simulink subsystem "Transmitter"  (R2022b)
settings: Solver=VariableStepAuto  StartTime=0.0  StopTime=10.0  RelTol=1e-3
undefined symbols (not defined in the file or in its folder): debugHeaderGain, G, Rsym
libraries: simulink x44, hdlsllib x29, dspsigops x7, dsphdlfiltering2 x1, whdlmod x1
(part 1 of 2)
settings Model: Creator=svdvl  LastModifiedBy=svdvl

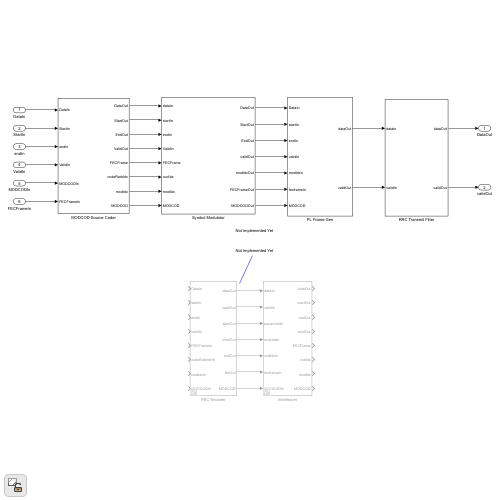
[thumbnail: Simulink's stored preview of the top-level diagram]
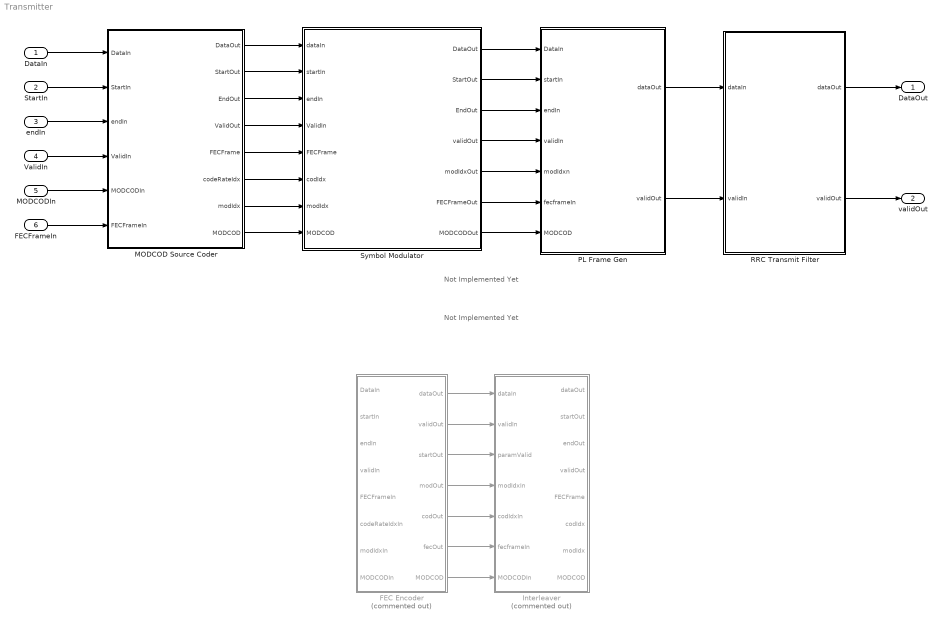
== system Transmitter ==
  note: Not Implemented Yet
  note: Not Implemented Yet
  DataIn : Inport
  StartIn : Inport  Port=2
  endIn : Inport  Port=3
  ValidIn : Inport  Port=4
  MODCODIn : Inport  Port=5
  FECFrameIn : Inport  Port=6
  FEC Encoder : Subsystem  Commented=on
  Interleaver : Subsystem  Commented=on
  MODCOD Source Coder : Subsystem
  PL Frame Gen : Subsystem
  RRC Transmit Filter : Subsystem
  Symbol Modulator : Subsystem
  DataOut : Outport
  validOut : Outport  Port=2
  wires:
  RRC Transmit Filter/2(validOut) -> validOut/1
  RRC Transmit Filter/1(dataOut) -> DataOut/1
  MODCOD Source Coder/5(FECFrame) -> Symbol Modulator/5(FECFrame)
  MODCOD Source Coder/3(EndOut) -> Symbol Modulator/3(endIn)
  MODCOD Source Coder/8(MODCOD) -> Symbol Modulator/8(MODCOD)
  MODCOD Source Coder/6(codeRateIdx) -> Symbol Modulator/6(codIdx)
  MODCOD Source Coder/4(ValidOut) -> Symbol Modulator/4(ValidIn)
  MODCOD Source Coder/2(StartOut) -> Symbol Modulator/2(startIn)
  MODCOD Source Coder/1(DataOut) -> Symbol Modulator/1(dataIn)
  Symbol Modulator/6(FECFrameOut) -> PL Frame Gen/6(fecframeIn)
  MODCOD Source Coder/7(modIdx) -> Symbol Modulator/7(modIdx)
  endIn/1 -> MODCOD Source Coder/3(endIn)
  Symbol Modulator/2(StartOut) -> PL Frame Gen/2(startIn)
  Symbol Modulator/7(MODCODOut) -> PL Frame Gen/7(MODCOD)
  StartIn/1 -> MODCOD Source Coder/2(StartIn)
  FECFrameIn/1 -> MODCOD Source Coder/6(FECFrameIn)
  PL Frame Gen/1(dataOut) -> RRC Transmit Filter/1(dataIn)
  DataIn/1 -> MODCOD Source Coder/1(DataIn)
  MODCODIn/1 -> MODCOD Source Coder/5(MODCODIn)
  Symbol Modulator/3(EndOut) -> PL Frame Gen/3(endIn)
  Symbol Modulator/5(modIdxOut) -> PL Frame Gen/5(modIdxn)
  Symbol Modulator/1(DataOut) -> PL Frame Gen/1(DataIn)
  Symbol Modulator/4(validOut) -> PL Frame Gen/4(validIn)
  PL Frame Gen/2(validOut) -> RRC Transmit Filter/2(validIn)
  ValidIn/1 -> MODCOD Source Coder/4(ValidIn)
  FEC Encoder/7(MODCOD) -> Interleaver/7(MODCODIn)
  FEC Encoder/1(dataOut) -> Interleaver/1(dataIn)
  FEC Encoder/4(modOut) -> Interleaver/4(modIdxIn)
  FEC Encoder/5(codOut) -> Interleaver/5(codIdxIn)
  FEC Encoder/3(startOut) -> Interleaver/3(paramValid)
  FEC Encoder/2(validOut) -> Interleaver/2(validIn)
  FEC Encoder/6(fecOut) -> Interleaver/6(fecframeIn)

== system Transmitter/FEC Encoder ==
  DataIn : Inport
  startIn : Inport  Port=2
  endIn : Inport  Port=3
  validIn : Inport  Port=4
  FECFrameIn : Inport  Port=5
  codeRateIdxIn : Inport  Port=6
  modIdxIn : Inport  Port=7
  MODCODIn : Inport  Port=8
  Terminator : Terminator
  dataOut : Outport
  validOut : Outport  Port=2
  startOut : Outport  Port=3
  modOut : Outport  Port=4
  codOut : Outport  Port=5
  fecOut : Outport  Port=6
  MODCOD : Outport  Port=7
  wires:
  DataIn/1 -> dataOut/1
  startIn/1 -> startOut/1
  modIdxIn/1 -> modOut/1
  codeRateIdxIn/1 -> codOut/1
  FECFrameIn/1 -> fecOut/1
  MODCODIn/1 -> MODCOD/1
  validIn/1 -> validOut/1
  endIn/1 -> Terminator/1

== system Transmitter/Interleaver ==
  dataIn : Inport
  validIn : Inport  Port=2
  paramValid : Inport  Port=3
  modIdxIn : Inport  Port=4
  codIdxIn : Inport  Port=5
  fecframeIn : Inport  Port=6
  MODCODIn : Inport  Port=7
  dataOut : Outport
  startOut : Outport  Port=2
  endOut : Outport  Port=3
  validOut : Outport  Port=4
  FECFrame : Outport  Port=5
  codIdx : Outport  Port=6
  modIdx : Outport  Port=7
  MODCOD : Outport  Port=8
  wires:
  dataIn/1 -> dataOut/1
  validIn/1 -> validOut/1

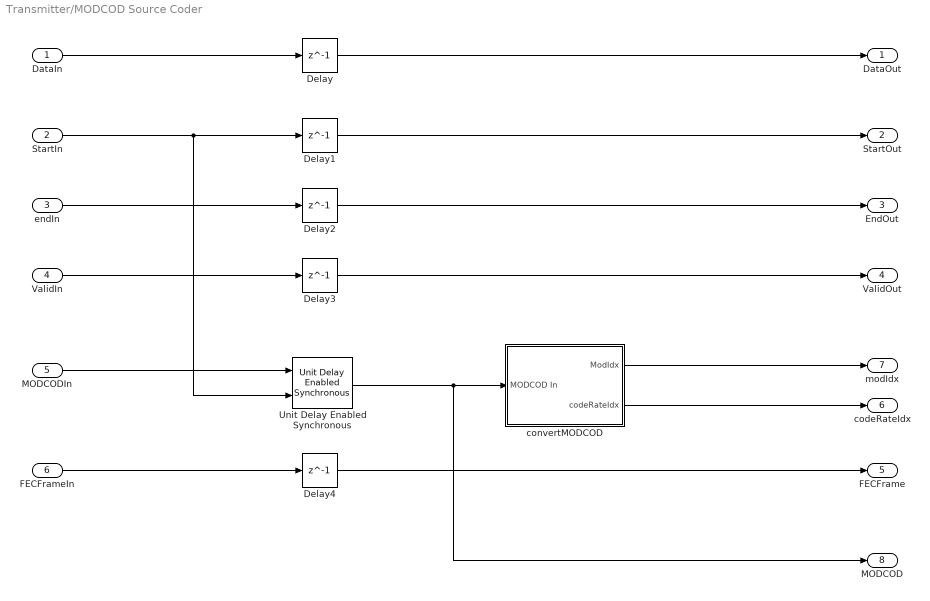
== system Transmitter/MODCOD Source Coder ==
  DataIn : Inport
  StartIn : Inport  Port=2
  endIn : Inport  Port=3
  ValidIn : Inport  Port=4
  MODCODIn : Inport  Port=5
  FECFrameIn : Inport  Port=6
  Delay{,1..4} (5 alike) : Delay  DelayLength=1
  Unit Delay Enabled Synchronous : hdlsllib/Discrete/Unit Delay Enabled Synchronous  InitialCondition=0.0  SampleTime=-1
  convertMODCOD : Subsystem
  DataOut : Outport
  StartOut : Outport  Port=2
  EndOut : Outport  Port=3
  ValidOut : Outport  Port=4
  FECFrame : Outport  Port=5
  codeRateIdx : Outport  Port=6
  modIdx : Outport  Port=7
  MODCOD : Outport  Port=8
  wires:
  MODCODIn/1 -> Unit Delay Enabled Synchronous/1
  DataIn/1 -> Delay/1
  StartIn/1 -> Unit Delay Enabled Synchronous/2, Delay1/1
  endIn/1 -> Delay2/1
  ValidIn/1 -> Delay3/1
  Unit Delay Enabled Synchronous/1 -> convertMODCOD/1(MODCOD In), MODCOD/1
  convertMODCOD/1(ModIdx) -> modIdx/1
  convertMODCOD/2(codeRateIdx) -> codeRateIdx/1
  FECFrameIn/1 -> Delay4/1
  Delay/1 -> DataOut/1
  Delay1/1 -> StartOut/1
  Delay2/1 -> EndOut/1
  Delay3/1 -> ValidOut/1
  Delay4/1 -> FECFrame/1

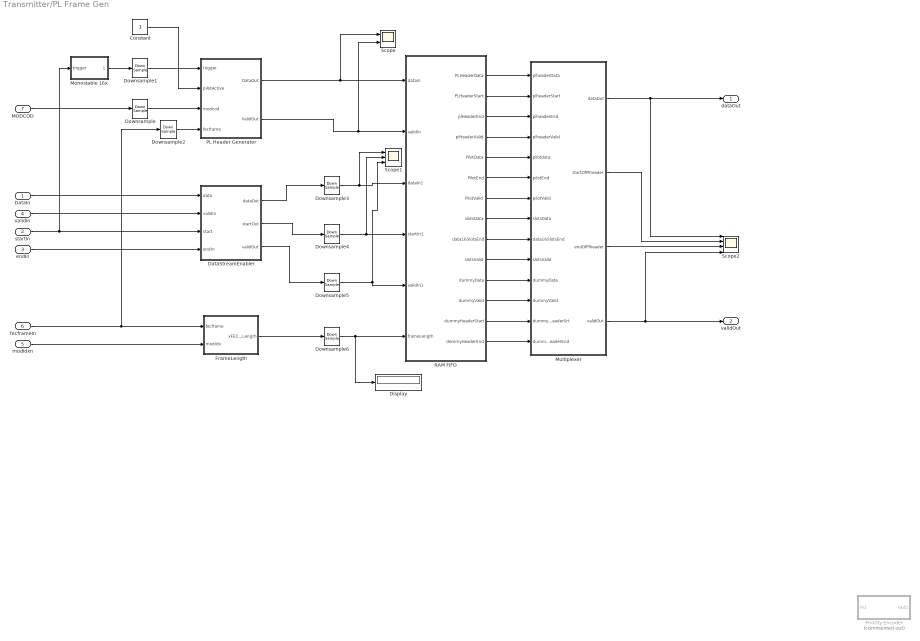
== system Transmitter/PL Frame Gen ==
  DataIn : Inport
  startIn : Inport  Port=2
  endIn : Inport  Port=3
  validIn : Inport  Port=4
  modIdxn : Inport  Port=5
  fecframeIn : Inport  Port=6
  MODCOD : Inport  Port=7
  Constant : Constant  OutDataTypeStr=boolean  SampleTime=2/Rsym
  DataStreamEnabler : Subsystem
  Display : Display
  Downsample : DownSample  N=16  RateOptions=Allow multirate processing
  Downsample1 : DownSample  N=16  RateOptions=Allow multirate processing
  Downsample2 : DownSample  N=16  RateOptions=Allow multirate processing
  Downsample{3..6} (4 alike) : DownSample  N=8  RateOptions=Allow multirate processing
  FrameLength : Subsystem
  Monostable 16x : Subsystem
  Multiplexer : Subsystem
  PL Header Generator : Subsystem
  Priority Encoder : Subsystem  Commented=on
  RAM FIFO : Subsystem
  Scope : Scope  NumInputPorts=2
  Scope1 : Scope  NumInputPorts=3
  Scope2 : Scope  NumInputPorts=4
  dataOut : Outport
  validOut : Outport  Port=2
  wires:
  MODCOD/1 -> Downsample/1
  Downsample/1 -> PL Header Generator/3(modcod)
  startIn/1 -> DataStreamEnabler/3(start), Monostable 16x/1(trigger)
  DataIn/1 -> DataStreamEnabler/1(data)
  validIn/1 -> DataStreamEnabler/2(validIn)
  endIn/1 -> DataStreamEnabler/4(endIn)
  fecframeIn/1 -> Downsample2/1, FrameLength/1(fecframe)
  modIdxn/1 -> FrameLength/2(modIdx)
  Downsample1/1 -> PL Header Generator/1(trigger)
  Downsample2/1 -> PL Header Generator/4(fecframe)
  DataStreamEnabler/1(dataOut) -> Downsample3/1
  DataStreamEnabler/2(startOut) -> Downsample4/1
  DataStreamEnabler/3(validOut) -> Downsample5/1
  FrameLength/1(xFECFrameLength) -> Downsample6/1
  Constant/1 -> PL Header Generator/2(pilotActive)
  Downsample6/1 -> Display/1, RAM FIFO/6(frameLength)
  PL Header Generator/1(DataOut) -> Scope/1, RAM FIFO/1(dataIn)
  PL Header Generator/2(ValidOut) -> Scope/2, RAM FIFO/2(validIn)
  Downsample3/1 -> Scope1/1, RAM FIFO/3(dataIn1)
  Downsample4/1 -> Scope1/2, RAM FIFO/4(startIn1)
  Downsample5/1 -> Scope1/3, RAM FIFO/5(validIn1)
  Monostable 16x/1(validOut) -> Downsample1/1
  RAM FIFO/1(PLHeaderData) -> Multiplexer/1(plheaderData)
  RAM FIFO/2(PLHeaderStart) -> Multiplexer/2(plheaderStart)
  RAM FIFO/3(plHeaderEnd) -> Multiplexer/3(plheaderEnd)
  RAM FIFO/4(plHeaderValid) -> Multiplexer/4(plheaderValid)
  RAM FIFO/5(PilotData) -> Multiplexer/5(pilotdata)
  RAM FIFO/6(PilotEnd) -> Multiplexer/6(pilotEnd)
  RAM FIFO/7(PilotValid) -> Multiplexer/7(pilotValid)
  RAM FIFO/8(slotsData) -> Multiplexer/8(slotsData)
  RAM FIFO/9(data16SlotsEnd) -> Multiplexer/9(data16SlotsEnd)
  RAM FIFO/10(slotsValid) -> Multiplexer/10(slotsValid)
  RAM FIFO/11(dummyData) -> Multiplexer/11(dummyData)
  RAM FIFO/12(dummyValid) -> Multiplexer/12(dummyValid)
  RAM FIFO/13(dummyHeaderStart) -> Multiplexer/13(dummyHeaderSrt)
  RAM FIFO/14(demmyHeaderEnd) -> Multiplexer/14(dummyHeaderEnd)
  Multiplexer/1(dataOut) -> dataOut/1, Scope2/1
  Multiplexer/2(startOfPlheader) -> Scope2/2
  Multiplexer/3(endOfPlheader) -> Scope2/3
  Multiplexer/4(validOut) -> validOut/1, Scope2/4

== system Transmitter/RRC Transmit Filter ==
  dataIn : Inport
  validIn : Inport  Port=2
  Discrete FIR Filter : dsphdlfiltering2/Discrete FIR Filter  NumeratorSource=Property  Numerator="[-0.00285820997079789\t0.00137733032508190\t0.00315455482520775\t-0.00356415296709377\t-0.00206211933009069\t0.00514477794743620\t-0.000825518525453186\t-0.00481272795526686\t0.00560922270003514\t0.000910808542107733\t-0.0120044818773511\t0.00862996822246556\t0.0193455321229390\t-0.0268242332250627\t-0.0266806119948057\t0.0600224093867556\t0.0329422984385442\t-0.130628932045810\t-0.0371565869289195\t0.443442194227448\t0.745765109300838\t0.443442194227448\t-0.0371565869289195\t-0.130628932045810\t0.0329422984385442\t0.0600224093867556\t-0.0266806119948057\t-0.0268242332250627\t0.0193455321229390\t0.00862996822246556\t-0.0120044818773511\t0.000910808542107733\t0.00560922270003514\t-0.00481272795526686\t-0.000825518525453186\t0.00514477794743620\t-0.00206211933009069\t-0.00356415296709377\t0.00315455482520775\t0.00137733032508190\t-0.00285820997079789]"  NumeratorPrototype=[]  FilterStructure=Direct form systolic  SerializationOption=Minimum number of cycles between valid input samples  NumCycles=2  NumberOfMultipliers=2  SimulateUsing=Code generation  roundingMode=Floor  overflowMode=off  CoefficientsDataTypeStr=Inherit: Same word length as input  OutputDataTypeStr=Inherit: Same word length as input  ResetInputPort=off  HDLGlobalReset=off
  Repeat : dspsigops/Repeat  N=2  RateOptions=Allow multirate processing  ic=0  mode=Unused parameter value
      settings: LibrarySourceBlock=dsphdlsupportsigops/Repeat
  Upsample : dspsigops/Upsample  N=2  phase=0  RateOptions=Allow multirate processing  ic=0  mode=Unused parameter value
      settings: LibrarySourceBlock=dsphdlsupportsigops/Upsample
  dataOut : Outport
  validOut : Outport  Port=2
  wires:
  dataIn/1 -> Upsample/1
  Discrete FIR Filter/1 -> dataOut/1
  Discrete FIR Filter/2 -> validOut/1
  validIn/1 -> Repeat/1
  Upsample/1 -> Discrete FIR Filter/1
  Repeat/1 -> Discrete FIR Filter/2

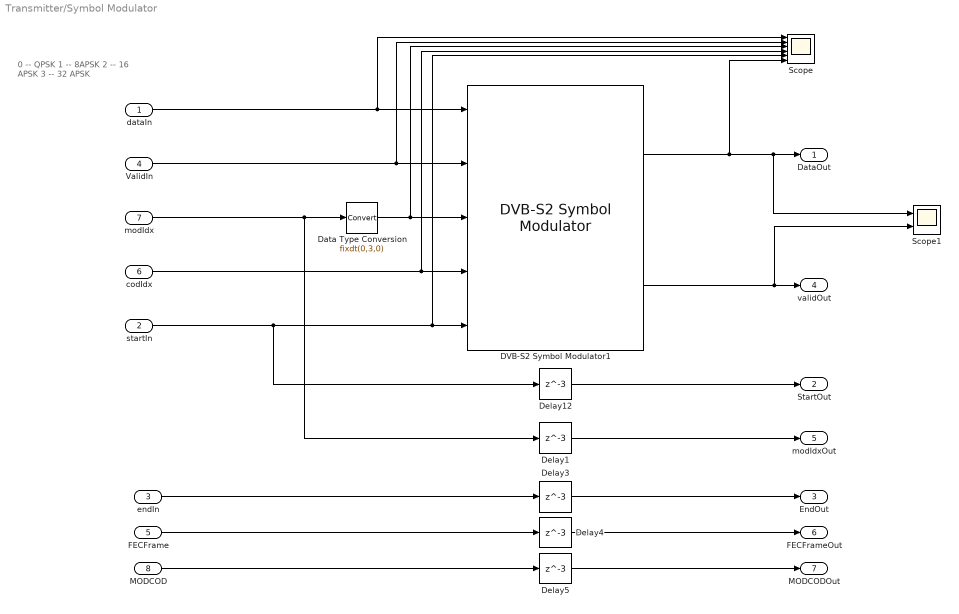
== system Transmitter/Symbol Modulator ==
  note: 0 -- QPSK
      | 1 -- 8APSK
      | 2 -- 16 APSK
      | 3 -- 32 APSK
  dataIn : Inport
  startIn : Inport  Port=2
  endIn : Inport  Port=3
  ValidIn : Inport  Port=4
  FECFrame : Inport  Port=5
  codIdx : Inport  Port=6
  modIdx : Inport  Port=7
  MODCOD : Inport  Port=8
  DVB-S2 Symbol Modulator1 : whdlmod/DVB-S2 Symbol Modulator  ModulationSourceParams=Input port  ModulationScheme=QPSK  CodeRateAPSK=3/4  UnitAveragePower=on  SimulateUsing=Code generation  OutputDataType=double  WordLength=18
  Data Type Conversion : DataTypeConversion  OutDataTypeStr=fixdt(0,3,0)  SaturateOnIntegerOverflow=off  RndMeth=Floor
  Delay{1,3..5,12} (5 alike) : Delay  DelayLength=3
  Scope : Scope  NumInputPorts=6
  Scope1 : Scope  NumInputPorts=2
  DataOut : Outport
  StartOut : Outport  Port=2
  EndOut : Outport  Port=3
  validOut : Outport  Port=4
  modIdxOut : Outport  Port=5
  FECFrameOut : Outport  Port=6
  MODCODOut : Outport  Port=7
  wires:
  dataIn/1 -> Scope/1, DVB-S2 Symbol Modulator1/1
  ValidIn/1 -> Scope/2, DVB-S2 Symbol Modulator1/2
  modIdx/1 -> Delay1/1, Data Type Conversion/1
  codIdx/1 -> Scope/4, DVB-S2 Symbol Modulator1/4
  startIn/1 -> Delay12/1, Scope/5, DVB-S2 Symbol Modulator1/5
  Data Type Conversion/1 -> Scope/3, DVB-S2 Symbol Modulator1/3
  DVB-S2 Symbol Modulator1/1 -> Scope/6, Scope1/1, DataOut/1
  DVB-S2 Symbol Modulator1/2 -> Scope1/2, validOut/1
  FECFrame/1 -> Delay4/1
  MODCOD/1 -> Delay5/1
  endIn/1 -> Delay3/1
  Delay12/1 -> StartOut/1
  Delay1/1 -> modIdxOut/1
  Delay3/1 -> EndOut/1
  Delay4/1 -> FECFrameOut/1
  Delay5/1 -> MODCODOut/1

== system Transmitter/MODCOD Source Coder/convertMODCOD ==
  note: 0 -- 1/4
      | 1 -- 1/3
      | 2 -- 2/5
      | 3 -- 1/2
      | 4 -- 3/5
      | 5 -- 2/3
      | 6 -- 3/4
      | 7 -- 4/5
      | 8 -- 5/6
      | 9 -- 8/9
      | 10 -- 9/10
  note: 0 -- QPSK
      | 1 -- 8APSK
      | 2 -- 16 APSK
      | 3 -- 32 APSK
  note: MODCOD DVB-S2
      | 1-11 QPSK
      | 2-17 8APSK
      | 18-23 16 APSK
      | 24-28 32 APSK
      | 29 QPSK (1/2) NEW
      | 29-31 RESERVED
      | 32 DUMMY
  MODCOD In : Inport
  1-D Lookup Table : Lookup_n-D  NumberOfTableDimensions=1  BreakpointsSpecification=Even spacing  BreakpointsForDimension1=[1:29]  Table=[0, 1, 2, 3, 4, 5, 6, 7, 8, 9, 10, 4, 5, 6, 8, 9, 10, 5, 6, 7, 8, 9, 10, 6, 7, 8, 9, 10, 3]  ExtrapMethod=Clip  UseLastTableValue=on  InternalRulePriority=Speed  OutDataTypeStr=fixdt(0, 4, 0)  RndMeth=Simplest
  Compare To Constant : simulink/Logic and Bit Operations/Compare To Constant  relop=<  const=12  OutDataTypeStr=boolean
  Compare To Constant1 : simulink/Logic and Bit Operations/Compare To Constant  relop=<  const=18  OutDataTypeStr=boolean
  Compare To Constant2 : simulink/Logic and Bit Operations/Compare To Constant  relop=<  const=24  OutDataTypeStr=boolean
  Compare To Constant3 : simulink/Logic and Bit Operations/Compare To Constant  relop===  const=29  OutDataTypeStr=boolean
  Constant : Constant  Value=0  OutDataTypeStr=fixdt(0,3,0)  SampleTime=-1
  Constant1 : Constant  OutDataTypeStr=fixdt(0,3,0)  SampleTime=-1
  Constant2 : Constant  Value=2  OutDataTypeStr=fixdt(0,3,0)  SampleTime=-1
  Constant3 : Constant  Value=3  OutDataTypeStr=fixdt(0,3,0)  SampleTime=-1
  Logical Operator : Logic  Operator=OR  AllPortsSameDT=off  OutDataTypeStr=boolean
  Scope : Scope  NumInputPorts=2
  Switch : Switch  Criteria=u2 ~= 0  SaturateOnIntegerOverflow=off  InputSameDT=off
  Switch1 : Switch  Criteria=u2 ~= 0  SaturateOnIntegerOverflow=off  InputSameDT=off
  Switch2 : Switch  Criteria=u2 ~= 0  SaturateOnIntegerOverflow=off  InputSameDT=off
  ModIdx : Outport
  codeRateIdx : Outport  Port=2
  wires:
  Constant3/1 -> Switch2/3
  Compare To Constant/1 -> Switch/2
  Constant1/1 -> Switch1/1
  Compare To Constant1/1 -> Switch1/2
  Switch/1 -> Scope/1, ModIdx/1
  MODCOD In/1 -> Compare To Constant1/1, Compare To Constant/1, Compare To Constant3/1, 1-D Lookup Table/1, Compare To Constant2/1
  Constant/1 -> Switch/1
  Constant2/1 -> Switch2/1
  Switch2/1 -> Switch1/3
  Switch1/1 -> Switch/3
  1-D Lookup Table/1 -> Scope/2, codeRateIdx/1
  Compare To Constant2/1 -> Logical Operator/1
  Compare To Constant3/1 -> Logical Operator/2
  Logical Operator/1 -> Switch2/2

== system Transmitter/PL Frame Gen/DataStreamEnabler ==
  data : Inport
  validIn : Inport  Port=2
  start : Inport  Port=3
  endIn : Inport  Port=4
  Scope : Scope  NumInputPorts=3
  Unit Delay Enabled Synchronous : hdlsllib/Discrete/Unit Delay Enabled Synchronous  InitialCondition=0.0  SampleTime=-1
  monostable 8x : Subsystem
  dataOut : Outport
  startOut : Outport  Port=2
  validOut : Outport  Port=3
  wires:
  data/1 -> Unit Delay Enabled Synchronous/1
  validIn/1 -> Unit Delay Enabled Synchronous/2
  Unit Delay Enabled Synchronous/1 -> Scope/1, dataOut/1
  start/1 -> monostable 8x/1(startIn)
  endIn/1 -> monostable 8x/2(endIn)
  monostable 8x/1(startOut) -> Scope/2, startOut/1
  monostable 8x/2(ValidOut) -> Scope/3, validOut/1

== system Transmitter/PL Frame Gen/FrameLength ==
  note: Number of symbols in a frame
  note: 0 normal frame
      | 1 short frame
      | 2 medium frame
  note: modIdx encodes the number of bits in a symbol
      | 0 -- 2 bits per constellation point
      | 1 -- 3 bits
      | 2 -- 4 bits
      | 3 -- 5 bits
      | 4 -- 6 bits
  fecframe : Inport
  modIdx : Inport  Port=2
  Display : Display
  Display1 : Display
  Display2 : Display
  Medium Frame xFECFrame Length1 : Lookup_n-D  NumberOfTableDimensions=1  BreakpointsSpecification=Even spacing  BreakpointsForDimension1=[-5:5]  BreakpointsForDimension1FirstPoint=0  Table=32400./log2([4 8 16 32 64])  TableDataTypeStr=fixdt(0,15,0)  InterpMethod=Flat  InternalRulePriority=Speed  OutDataTypeStr=fixdt(0,15,0)  RndMeth=Simplest
  Multiport Switch : MultiPortSwitch  DataPortOrder=Zero-based contiguous  zeroidx=on  SaturateOnIntegerOverflow=off  InputSameDT=off
  Normal Frame xFECFrame Length : Lookup_n-D  NumberOfTableDimensions=1  BreakpointsSpecification=Even spacing  BreakpointsForDimension1=[-5:5]  BreakpointsForDimension1FirstPoint=0  Table=64800./log2([4 8 16 32 64])  TableDataTypeStr=fixdt(0,15,0)  InterpMethod=Flat  InternalRulePriority=Speed  OutDataTypeStr=fixdt(0,15,0)  RndMeth=Simplest
  Short Frame xFECFrame Length : Lookup_n-D  NumberOfTableDimensions=1  BreakpointsSpecification=Even spacing  BreakpointsForDimension1=[-5:5]  BreakpointsForDimension1FirstPoint=0  Table=16200./log2([4 8 16 32 64])  TableDataTypeStr=fixdt(0,15,0)  InterpMethod=Flat  InternalRulePriority=Speed  OutDataTypeStr=fixdt(0,15,0)  RndMeth=Simplest
  xFECFrameLength : Outport
  wires:
  fecframe/1 -> Multiport Switch/1, Display/1
  Normal Frame xFECFrame Length/1 -> Multiport Switch/2
  Multiport Switch/1 -> xFECFrameLength/1, Display1/1
  modIdx/1 -> Medium Frame xFECFrame Length1/1, Short Frame xFECFrame Length/1, Normal Frame xFECFrame Length/1, Display2/1
  Medium Frame xFECFrame Length1/1 -> Multiport Switch/4
  Short Frame xFECFrame Length/1 -> Multiport Switch/3

== system Transmitter/PL Frame Gen/Monostable 16x ==
  trigger : Inport
  Compare To Constant : simulink/Logic and Bit Operations/Compare To Constant  relop===  const=16  OutDataTypeStr=boolean
  Compare To Constant1 : simulink/Logic and Bit Operations/Compare To Constant  relop=~=  const=0  OutDataTypeStr=boolean
  HDL Counter : hdlsllib/Sources/HDL Counter  CountType=Count limited  CountInit=0  CountStep=1  CountMax=16  CountFromType=Initial value  CountFrom=0  CountResetPort=on  CountLoadPort=off  CountEnbPort=on  CountDirPort=off  CountHitOutputPort=off  CountDataType=Unsigned  CountWordLen=8  CountFracLen=0  CountSampTime=1
  Logical Operator : Logic  Operator=OR  AllPortsSameDT=off  OutDataTypeStr=boolean
  Scope : Scope  NumInputPorts=3
  validOut : Outport
  wires:
  HDL Counter/1 -> Scope/1, Compare To Constant1/1, Compare To Constant/1
  trigger/1 -> Logical Operator/1
  Logical Operator/1 -> Scope/2, HDL Counter/2
  Compare To Constant/1 -> HDL Counter/1, Scope/3
  Compare To Constant1/1 -> Logical Operator/2, validOut/1

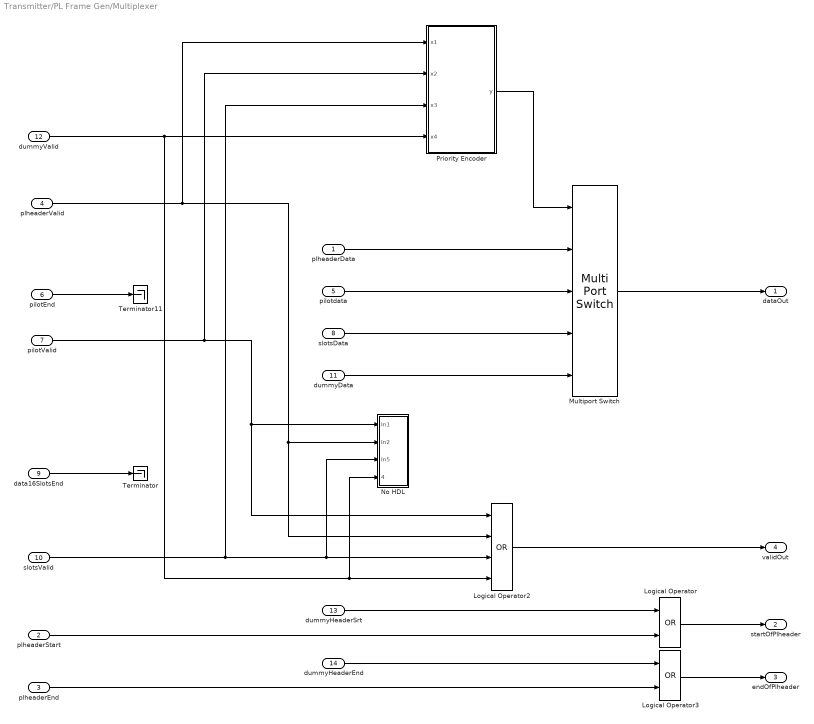
== system Transmitter/PL Frame Gen/Multiplexer ==
  plheaderData : Inport
  plheaderStart : Inport  Port=2
  plheaderEnd : Inport  Port=3
  plheaderValid : Inport  Port=4
  pilotdata : Inport  Port=5
  pilotEnd : Inport  Port=6
  pilotValid : Inport  Port=7
  slotsData : Inport  Port=8
  data16SlotsEnd : Inport  Port=9
  slotsValid : Inport  Port=10
  dummyData : Inport  Port=11
  dummyValid : Inport  Port=12
  dummyHeaderSrt : Inport  Port=13
  dummyHeaderEnd : Inport  Port=14
  Logical Operator : Logic  Operator=OR  AllPortsSameDT=off  OutDataTypeStr=boolean
  Logical Operator2 : Logic  Operator=OR  Inputs=4  AllPortsSameDT=off  OutDataTypeStr=boolean
  Logical Operator3 : Logic  Operator=OR  AllPortsSameDT=off  OutDataTypeStr=boolean
  Multiport Switch : MultiPortSwitch  DataPortOrder=Zero-based contiguous  Inputs=4  zeroidx=on  SaturateOnIntegerOverflow=off  InputSameDT=off
  No HDL : Subsystem
  Priority Encoder : MATLAB Function  TreatAsAtomicUnit=on
  Terminator : Terminator
  Terminator11 : Terminator
  dataOut : Outport
  startOfPlheader : Outport  Port=2
  endOfPlheader : Outport  Port=3
  validOut : Outport  Port=4
  wires:
  slotsValid/1 -> Priority Encoder/3(x3), No HDL/3(In5), Logical Operator2/3
  pilotValid/1 -> Priority Encoder/2(x2), Logical Operator2/1, No HDL/1(In1)
  data16SlotsEnd/1 -> Terminator/1
  plheaderValid/1 -> Priority Encoder/1(x1), Logical Operator2/2, No HDL/2(In2)
  pilotEnd/1 -> Terminator11/1
  Logical Operator2/1 -> validOut/1
  plheaderStart/1 -> Logical Operator/2
  dummyValid/1 -> No HDL/4(dummyValid), Logical Operator2/4, Priority Encoder/4(x4)
  Priority Encoder/1(y) -> Multiport Switch/1
  Multiport Switch/1 -> dataOut/1
  plheaderEnd/1 -> Logical Operator3/2
  plheaderData/1 -> Multiport Switch/2
  pilotdata/1 -> Multiport Switch/3
  slotsData/1 -> Multiport Switch/4
  dummyData/1 -> Multiport Switch/5
  dummyHeaderSrt/1 -> Logical Operator/1
  dummyHeaderEnd/1 -> Logical Operator3/1
  Logical Operator/1 -> startOfPlheader/1
  Logical Operator3/1 -> endOfPlheader/1

== system Transmitter/PL Frame Gen/PL Header Generator ==
  note: 1 at the start of the frame, else zero
  trigger : Inport
  pilotActive : Inport  Port=2
  modcod : Inport  Port=3
  fecframe : Inport  Port=4
  PL Header Bits Generator : Subsystem
  Terminator : Terminator
  Terminator1 : Terminator
  pi2 BSPK Modulator : Subsystem
  DataOut : Outport
  ValidOut : Outport  Port=2
  wires:
  modcod/1 -> PL Header Bits Generator/3(modcod)
  fecframe/1 -> PL Header Bits Generator/4(fecframe)
  pilotActive/1 -> PL Header Bits Generator/2(pilotActive)
  PL Header Bits Generator/1(bitsOut) -> pi2 BSPK Modulator/1(bitsIn)
  PL Header Bits Generator/5(UnscrambledBits) -> Terminator1/1
  PL Header Bits Generator/2(bitsStart) -> pi2 BSPK Modulator/2(startIn)
  PL Header Bits Generator/3(bitsEnd) -> Terminator/1
  PL Header Bits Generator/4(bitsValid) -> pi2 BSPK Modulator/3(validIn)
  trigger/1 -> PL Header Bits Generator/1(trigger)
  pi2 BSPK Modulator/1(dataOut) -> DataOut/1
  pi2 BSPK Modulator/2(validOut) -> ValidOut/1

== system Transmitter/PL Frame Gen/Priority Encoder ==
  In1 : Inport
  Out1 : Outport
  wires:
  In1/1 -> Out1/1

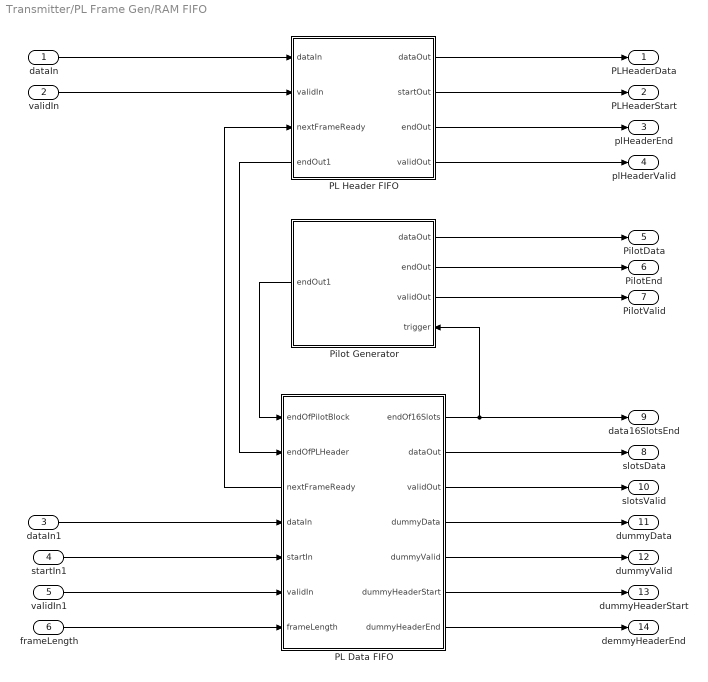
== system Transmitter/PL Frame Gen/RAM FIFO ==
  dataIn : Inport
  validIn : Inport  Port=2
  dataIn1 : Inport  Port=3
  startIn1 : Inport  Port=4
  validIn1 : Inport  Port=5
  frameLength : Inport  Port=6
  PL Data FIFO : Subsystem
      settings: PortSchema="{\"entries\":[{\"content\":{\"sides\":[{\"content\":{\"connectorIds\":[\"In1\",\"In2\",\"Out8\",\"In3\",\"In4\",\"In5\",\"In6\"]},\"type\":\"ConnectorPlacement.EquallySpacedRectSide\",\"uuid\":\"25a34951-0e23-4521-a61b-dabf4b9336a4\"},{\"content\":{\"connectorIds\":[\"Out1\",\"Out2\",\"Out3\",\"Out4\",\"Out5\",\"Out6\",\"Out7\"],\"side\":\"RIGHT\"},\"type\":\"ConnectorPlacement.EquallySpacedRectSide\",\"uuid\":\"eec023cc-e680-48cd-aceb-aeed48d064f6\"},{\"content\":{\"connectorIds\":[],\"side\":\"TOP\"},\"type\":\"ConnectorPlacement.EquallySpacedRectSide\",\"uuid\":\"ba8535a0-f40b-4ae2-82de-dd038ee14b99\"}]},\"type\":\"ConnectorPlacement.EquallySpacedConnector\",\"uuid\":\"91f1fe09-1e9a-44d5-8ef2-9c0919c45888\"}],\"packageUris\":[\"http://schema.mathworks.com/mf0/Connector/R2020b\"],\"version\":\"1.0\"}"
  PL Header FIFO : Subsystem
      settings: PortSchema="{\"entries\":[{\"content\":{\"sides\":[{\"content\":{\"connectorIds\":[\"In1\",\"In2\",\"In3\",\"Out5\"]},\"type\":\"ConnectorPlacement.EquallySpacedRectSide\",\"uuid\":\"aafc3790-84d7-47f2-9fb1-8faf5993815a\"},{\"content\":{\"connectorIds\":[\"Out1\",\"Out2\",\"Out3\",\"Out4\"],\"side\":\"RIGHT\"},\"type\":\"ConnectorPlacement.EquallySpacedRectSide\",\"uuid\":\"84bad990-8305-4d8a-9017-b70768cb23df\"},{\"content\":{\"connectorIds\":[],\"side\":\"TOP\"},\"type\":\"ConnectorPlacement.EquallySpacedRectSide\",\"uuid\":\"718453a2-626e-4fdd-91b0-273e1ddff201\"}]},\"type\":\"ConnectorPlacement.EquallySpacedConnector\",\"uuid\":\"f39b9ed3-9da6-41f4-91dd-f38495849c59\"}],\"packageUris\":[\"http://schema.mathworks.com/mf0/Connector/R2020b\"],\"version\":\"1.0\"}"
  Pilot Generator : Subsystem
      settings: PortSchema="{\"entries\":[{\"content\":{\"sides\":[{\"content\":{\"connectorIds\":[\"Out4\"]},\"type\":\"ConnectorPlacement.EquallySpacedRectSide\",\"uuid\":\"706bcf59-d8ee-4989-91cf-ea4f25b7e8b9\"},{\"content\":{\"connectorIds\":[\"Out1\",\"Out2\",\"Out3\",\"In1\"],\"side\":\"RIGHT\"},\"type\":\"ConnectorPlacement.EquallySpacedRectSide\",\"uuid\":\"e51c253f-ddd6-4a98-807e-12bbbaaa1da6\"},{\"content\":{\"connectorIds\":[],\"side\":\"TOP\"},\"type\":\"ConnectorPlacement.EquallySpacedRectSide\",\"uuid\":\"735c13ec-e497-4f6e-bd46-68484c8ba86d\"},{\"content\":{\"connectorIds\":[],\"side\":\"BOTTOM\"},\"type\":\"ConnectorPlacement.EquallySpacedRectSide\",\"uuid\":\"c9c0922b-324d-4790-8d43-b5c0efaf1da1\"}]},\"type\":\"ConnectorPlacement.EquallySpacedConnector\",\"uuid\":\"8bfa05ab-9579-4880-ba6d-c6d7c25035aa\"}],\"packageUris\":[\"http://schema.mathworks.com/mf0/Connector/R2020b\"],\"version\":\"1.0\"}"
  PLHeaderData : Outport
  PLHeaderStart : Outport  Port=2
  plHeaderEnd : Outport  Port=3
  plHeaderValid : Outport  Port=4
  PilotData : Outport  Port=5
  PilotEnd : Outport  Port=6
  PilotValid : Outport  Port=7
  slotsData : Outport  Port=8
  data16SlotsEnd : Outport  Port=9
  slotsValid : Outport  Port=10
  dummyData : Outport  Port=11
  dummyValid : Outport  Port=12
  dummyHeaderStart : Outport  Port=13
  demmyHeaderEnd : Outport  Port=14
  wires:
  dataIn/1 -> PL Header FIFO/1(dataIn)
  validIn/1 -> PL Header FIFO/2(validIn)
  dataIn1/1 -> PL Data FIFO/3(dataIn)
  startIn1/1 -> PL Data FIFO/4(startIn)
  validIn1/1 -> PL Data FIFO/5(validIn)
  frameLength/1 -> PL Data FIFO/6(frameLength)
  PL Header FIFO/5(endOut1) -> PL Data FIFO/2(endOfPLHeader)
  PL Data FIFO/1(endOf16Slots) -> data16SlotsEnd/1, Pilot Generator/1(trigger)
  Pilot Generator/4(endOut1) -> PL Data FIFO/1(endOfPilotBlock)
  PL Data FIFO/8(nextFrameReady) -> PL Header FIFO/3(nextFrameReady)
  PL Data FIFO/7(dummyHeaderEnd) -> demmyHeaderEnd/1
  PL Data FIFO/6(dummyHeaderStart) -> dummyHeaderStart/1
  PL Data FIFO/5(dummyValid) -> dummyValid/1
  PL Data FIFO/4(dummyData) -> dummyData/1
  PL Data FIFO/3(validOut) -> slotsValid/1
  PL Data FIFO/2(dataOut) -> slotsData/1
  Pilot Generator/1(dataOut) -> PilotData/1
  Pilot Generator/2(endOut) -> PilotEnd/1
  Pilot Generator/3(validOut) -> PilotValid/1
  PL Header FIFO/4(validOut) -> plHeaderValid/1
  PL Header FIFO/3(endOut) -> plHeaderEnd/1
  PL Header FIFO/2(startOut) -> PLHeaderStart/1
  PL Header FIFO/1(dataOut) -> PLHeaderData/1

== system Transmitter/PL Frame Gen/DataStreamEnabler/monostable 8x ==
  startIn : Inport
  endIn : Inport  Port=2
  Constant : Constant  OutDataTypeStr=boolean  SampleTime=1/Rsym/8
  Logical Operator : Logic  Operator=XOR  AllPortsSameDT=off  OutDataTypeStr=boolean
  Resettable Delay : Delay  DelayLength=1  ExternalReset=Level  ShowEnablePort=on
      settings: InputPortMap=u0,e6,r5
  Scope : Scope  NumInputPorts=4
  Unit Delay : UnitDelay  SampleTime=-1  HasFrameUpgradeWarning=on
  monostable : Subsystem
  startOut : Outport
  ValidOut : Outport  Port=2
  wires:
  monostable/1(Out1) -> startOut/1
  startIn/1 -> monostable/1(In1), Resettable Delay/1, Scope/1
  endIn/1 -> Scope/4, Resettable Delay/3
  Constant/1 -> Logical Operator/1
  Logical Operator/1 -> Scope/2, Resettable Delay/2
  Resettable Delay/1 -> Scope/3, Unit Delay/1, ValidOut/1
  Unit Delay/1 -> Logical Operator/2

== system Transmitter/PL Frame Gen/Multiplexer/No HDL ==
  In1 : Inport
  In2 : Inport  Port=2
  In5 : Inport  Port=3
  dummyValid : Inport  Port=4
  Assertion : Assertion
  Assertion1 : Assertion
  Delay : Delay  DelayLength=5  InitialCondition=1
  Delay1 : Delay  DelayLength=5  InitialCondition=1
  Logical Operator{,1,3,5} (4 alike) : Logic  AllPortsSameDT=off  OutDataTypeStr=boolean
  Logical Operator2 : Logic  Operator=NOT  Inputs=3  AllPortsSameDT=off  OutDataTypeStr=boolean
  Logical Operator4 : Logic  Operator=OR  Inputs=3  AllPortsSameDT=off  OutDataTypeStr=boolean
  Logical Operator6 : Logic  Operator=NOT  AllPortsSameDT=off  OutDataTypeStr=boolean
  wires:
  In1/1 -> Logical Operator/1, Logical Operator1/1
  In5/1 -> Logical Operator1/2, Logical Operator3/2
  Logical Operator/1 -> Logical Operator4/1
  Logical Operator1/1 -> Logical Operator4/2
  Logical Operator3/1 -> Logical Operator4/3
  Logical Operator4/1 -> Logical Operator5/1, Logical Operator2/1
  In2/1 -> Logical Operator/2, Logical Operator3/1
  Logical Operator2/1 -> Delay/1
  dummyValid/1 -> Logical Operator5/2
  Logical Operator5/1 -> Logical Operator6/1
  Logical Operator6/1 -> Delay1/1
  Delay/1 -> Assertion/1
  Delay1/1 -> Assertion1/1

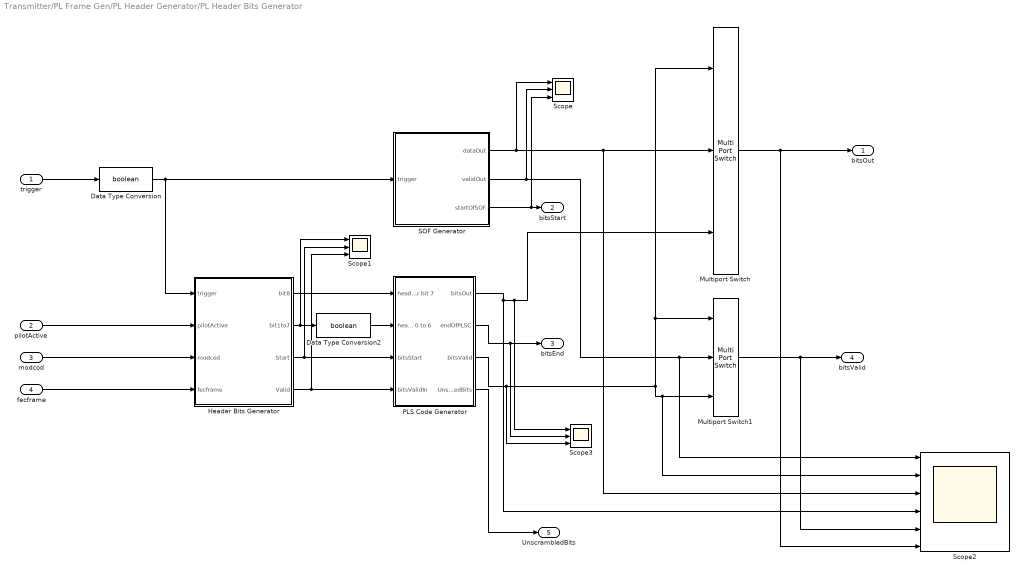
== system Transmitter/PL Frame Gen/PL Header Generator/PL Header Bits Generator ==
  trigger : Inport
  pilotActive : Inport  Port=2
  modcod : Inport  Port=3
  fecframe : Inport  Port=4
  Data Type Conversion : DataTypeConversion  OutDataTypeStr=boolean  SaturateOnIntegerOverflow=off  RndMeth=Floor
  Data Type Conversion2 : DataTypeConversion  OutDataTypeStr=boolean  SaturateOnIntegerOverflow=off  RndMeth=Floor
  Header Bits Generator : Subsystem
  Multiport Switch : MultiPortSwitch  DataPortOrder=Zero-based contiguous  Inputs=2  zeroidx=on  SaturateOnIntegerOverflow=off  InputSameDT=off
  Multiport Switch1 : MultiPortSwitch  DataPortOrder=Zero-based contiguous  Inputs=2  zeroidx=on  SaturateOnIntegerOverflow=off  InputSameDT=off
  PLS Code Generator : Subsystem
  SOF Generator : Subsystem
  Scope : Scope  NumInputPorts=3
  Scope1 : Scope  NumInputPorts=3
  Scope2 : Scope  NumInputPorts=6
  Scope3 : Scope  NumInputPorts=3
  bitsOut : Outport
  bitsStart : Outport  Port=2
  bitsEnd : Outport  Port=3
  bitsValid : Outport  Port=4
  UnscrambledBits : Outport  Port=5
  wires:
  SOF Generator/1(dataOut) -> Scope/1, Scope2/3, Multiport Switch/2
  Data Type Conversion/1 -> Header Bits Generator/1(trigger), SOF Generator/1(trigger)
  PLS Code Generator/1(bitsOut) -> Scope2/4, Scope3/1, Multiport Switch/3
  PLS Code Generator/3(bitsValid) -> Scope3/3, Multiport Switch1/1, Multiport Switch/1, Scope2/2, Multiport Switch1/3
  Multiport Switch/1 -> Scope2/6, bitsOut/1
  SOF Generator/3(startOfSOF) -> Scope/3, bitsStart/1
  PLS Code Generator/2(endOfPLSC) -> Scope3/2, bitsEnd/1
  SOF Generator/2(validOut) -> Scope/2, Scope2/1, Multiport Switch1/2
  Multiport Switch1/1 -> Scope2/5, bitsValid/1
  trigger/1 -> Data Type Conversion/1
  pilotActive/1 -> Header Bits Generator/2(pilotActive)
  modcod/1 -> Header Bits Generator/3(modcod)
  fecframe/1 -> Header Bits Generator/4(fecframe)
  Header Bits Generator/2(bit1to7) -> Scope1/1, Data Type Conversion2/1
  Header Bits Generator/3(Start) -> PLS Code Generator/3(bitsStart), Scope1/2
  Header Bits Generator/4(Valid) -> PLS Code Generator/4(bitsValidIn), Scope1/3
  PLS Code Generator/4(UnscrambledBits) -> UnscrambledBits/1
  Header Bits Generator/1(bit8) -> PLS Code Generator/1(header bit 7)
  Data Type Conversion2/1 -> PLS Code Generator/2(header bits 0 to 6)

== system Transmitter/PL Frame Gen/PL Header Generator/pi2 BSPK Modulator ==
  note: For debug purpose, to make the header noticable
  bitsIn : Inport
  startIn : Inport  Port=2
  validIn : Inport  Port=3
  Constant : Constant  Value=complex(0)  OutDataTypeStr=Inherit: Inherit via back propagation  SampleTime=-1
  Constant1 : Constant  Value=exp(-1i*3*pi/4)  OutDataTypeStr=fixdt(1,16,14)  SampleTime=-1
      mask init:
      | Simulink.suppressDiagnostic(gcb, 'SimulinkFixedPoint:util:fxpParameterPrecisionLoss');
  Constant2 : Constant  Value=exp(1i*pi/4)  OutDataTypeStr=fixdt(1,16,14)  SampleTime=-1
      mask init:
      | Simulink.suppressDiagnostic(gcb, 'SimulinkFixedPoint:util:fxpParameterPrecisionLoss');
  Data Type Conversion : DataTypeConversion  OutDataTypeStr=boolean  SaturateOnIntegerOverflow=off  RndMeth=Floor
  Delay4 : Delay  DelayLength=0
  Delay5 : Delay  DelayLength=1
  Extract Bits : simulink/Logic and Bit Operations/Extract Bits  bitsToExtract=Range of bits  numBits=8  bitIdxRange=0  outScalingMode=Treat bit field as an integer
  Gain : Gain  Gain=exp(1i*pi/2)  ParamDataTypeStr=fixdt(1,16,14)  OutDataTypeStr=Inherit: Same as input
      mask init:
      | Simulink.suppressDiagnostic(gcb, 'SimulinkFixedPoint:util:fxpParameterPrecisionLoss');
  HDL Counter : hdlsllib/Sources/HDL Counter  CountType=Count limited  CountInit=0  CountStep=1  CountMax=100  CountFromType=Initial value  CountFrom=0  CountResetPort=on  CountLoadPort=off  CountEnbPort=on  CountDirPort=off  CountHitOutputPort=off  CountDataType=Unsigned  CountWordLen=nextpow2(90 - 1)  CountFracLen=0  CountSampTime=1
  Multiply : Gain  Gain=debugHeaderGain  OutDataTypeStr=Inherit: Same as input
  Scope : Scope  NumInputPorts=3
  Switch : Switch  Criteria=u2 ~= 0  SaturateOnIntegerOverflow=off  InputSameDT=off
  Switch1 : Switch  Criteria=u2 ~= 0  SaturateOnIntegerOverflow=off  InputSameDT=off
  Switch2 : Switch  Criteria=u2 ~= 0  SaturateOnIntegerOverflow=off  InputSameDT=off
  dataOut : Outport
  validOut : Outport  Port=2
  wires:
  Multiply/1 -> dataOut/1
  Extract Bits/1 -> Data Type Conversion/1
  Gain/1 -> Switch1/1
  Delay4/1 -> HDL Counter/2, Switch2/2, validOut/1, Scope/2
  bitsIn/1 -> Scope/3, Delay5/1
  HDL Counter/1 -> Extract Bits/1
  validIn/1 -> Delay4/1
  startIn/1 -> HDL Counter/1
  Constant2/1 -> Switch/3
  Constant1/1 -> Switch/1
  Data Type Conversion/1 -> Switch1/2
  Delay5/1 -> Switch/2
  Switch/1 -> Switch1/3, Gain/1
  Switch1/1 -> Switch2/1, Scope/1
  Switch2/1 -> Multiply/1
  Constant/1 -> Switch2/3

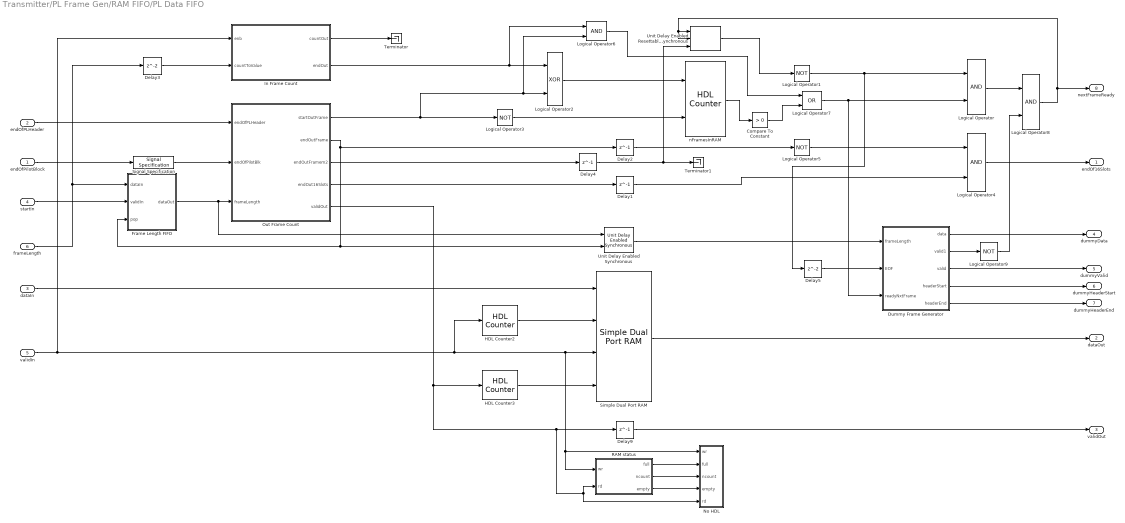
== system Transmitter/PL Frame Gen/RAM FIFO/PL Data FIFO ==
  endOfPilotBlock : Inport
  endOfPLHeader : Inport  Port=2
  dataIn : Inport  Port=3
  startIn : Inport  Port=4
  validIn : Inport  Port=5
  frameLength : Inport  Port=6
  Compare To Constant : simulink/Logic and Bit Operations/Compare To Constant  relop=>  const=0  OutDataTypeStr=boolean
  Delay{1..2,4,9} (4 alike) : Delay  DelayLength=1
  Delay3 : Delay
  Delay5 : Delay
  Dummy Frame Generator : Subsystem
  Frame Length FIFO : Subsystem
  HDL Counter2 : hdlsllib/Sources/HDL Counter  CountType=Count limited  CountInit=0  CountStep=1  CountMax=2^16-1  CountFromType=Initial value  CountFrom=0  CountResetPort=off  CountLoadPort=off  CountEnbPort=on  CountDirPort=off  CountHitOutputPort=off  CountDataType=Unsigned  CountWordLen=16  CountFracLen=0  CountSampTime=1
  HDL Counter3 : hdlsllib/Sources/HDL Counter  CountType=Count limited  CountInit=0  CountStep=1  CountMax=2^16-1  CountFromType=Initial value  CountFrom=0  CountResetPort=off  CountLoadPort=off  CountEnbPort=on  CountDirPort=off  CountHitOutputPort=off  CountDataType=Unsigned  CountWordLen=16  CountFracLen=0  CountSampTime=1
  In Frame Count : MATLAB Function  TreatAsAtomicUnit=on
  Logical Operator{,4,6,8} (4 alike) : Logic  AllPortsSameDT=off  OutDataTypeStr=boolean
  Logical Operator{1,3,5,9} (4 alike) : Logic  Operator=NOT  AllPortsSameDT=off  OutDataTypeStr=boolean
  Logical Operator2 : Logic  Operator=XOR  AllPortsSameDT=off  OutDataTypeStr=boolean
  Logical Operator7 : Logic  Operator=OR  AllPortsSameDT=off  OutDataTypeStr=boolean
  No HDL : Subsystem
  Out Frame Count : MATLAB Function  TreatAsAtomicUnit=on
  RAM status : MATLAB Function  TreatAsAtomicUnit=on
  Signal Specification : SignalSpecification  OutDataTypeStr=boolean
  Simple Dual Port RAM : hdlsllib/HDL RAMs/Simple Dual Port RAM  ram_size=16
  Terminator : Terminator
  Terminator1 : Terminator
  Unit Delay Enabled Synchronous : hdlsllib/Discrete/Unit Delay Enabled Synchronous  InitialCondition=0.0  SampleTime=-1
  Unit Delay Enabled Resettable Synchronous : hdlsllib/Discrete/Unit Delay Enabled Resettable Synchronous  InitialCondition=0.0  SampleTime=-1
  nFramesInRAM : hdlsllib/Sources/HDL Counter  CountType=Free running  CountInit=0  CountStep=1  CountMax=25  CountFromType=Initial value  CountFrom=0  CountResetPort=off  CountLoadPort=off  CountEnbPort=on  CountDirPort=on  CountHitOutputPort=off  CountDataType=Unsigned  CountWordLen=8  CountFracLen=0  CountSampTime=1
  endOf16Slots : Outport
  dataOut : Outport  Port=2
  validOut : Outport  Port=3
  dummyData : Outport  Port=4
  dummyValid : Outport  Port=5
  dummyHeaderStart : Outport  Port=6
  dummyHeaderEnd : Outport  Port=7
  nextFrameReady : Outport  Port=8
  wires:
  Out Frame Count/4(endOut16Slots) -> Delay1/1
  RAM status/3(empty) -> No HDL/4(empty)
  RAM status/2(ncount) -> No HDL/3(ncount)
  RAM status/1(full) -> No HDL/2(full)
  HDL Counter2/1 -> Simple Dual Port RAM/2
  Compare To Constant/1 -> Logical Operator7/2
  Logical Operator4/1 -> endOf16Slots/1
  Delay1/1 -> Logical Operator4/2
  endOfPilotBlock/1 -> Signal Specification/1
  Frame Length FIFO/1(dataOut) -> Unit Delay Enabled Synchronous/1, Out Frame Count/3(frameLength)
  Simple Dual Port RAM/1 -> dataOut/1
  Logical Operator3/1 -> nFramesInRAM/2
  Delay9/1 -> validOut/1
  Delay2/1 -> Logical Operator5/1
  Dummy Frame Generator/1(data) -> dummyData/1
  Logical Operator7/1 -> Logical Operator/2, Dummy Frame Generator/3(readyNxtFrame)
  Logical Operator1/1 -> Delay5/1, Logical Operator/1
  validIn/1 -> Simple Dual Port RAM/3, RAM status/1(wr), No HDL/1(wr), HDL Counter2/1, In Frame Count/1(enb)
  dataIn/1 -> Simple Dual Port RAM/1
  Logical Operator/1 -> Logical Operator8/1
  endOfPLHeader/1 -> Out Frame Count/1(endOfPLHeader)
  nFramesInRAM/1 -> Compare To Constant/1
  Dummy Frame Generator/3(valid) -> dummyValid/1
  Out Frame Count/1(startOutFrame) -> Logical Operator3/1, Logical Operator6/2, Logical Operator2/2
  Delay5/1 -> Dummy Frame Generator/2(EOF)
  Delay3/1 -> In Frame Count/2(countToValue)
  startIn/1 -> Frame Length FIFO/2(validIn)
  Delay4/1 -> Unit Delay Enabled Resettable Synchronous/3, Terminator1/1
  Dummy Frame Generator/2(valid1) -> Logical Operator9/1
  In Frame Count/2(endOut) -> Logical Operator6/1, Logical Operator2/1
  HDL Counter3/1 -> Simple Dual Port RAM/4
  Logical Operator2/1 -> nFramesInRAM/1
  Unit Delay Enabled Resettable Synchronous/1 -> Logical Operator1/1
  In Frame Count/1(countOut) -> Terminator/1
  Signal Specification/1 -> Out Frame Count/2(endOfPilotBlk)
  frameLength/1 -> Delay3/1, Frame Length FIFO/1(dataIn)
  Out Frame Count/5(validOut) -> Delay9/1, RAM status/2(rd), No HDL/5(rd), HDL Counter3/1
  Unit Delay Enabled Synchronous/1 -> Dummy Frame Generator/1(frameLength)
  Out Frame Count/2(endOutFrame) -> Frame Length FIFO/3(pop), Unit Delay Enabled Synchronous/2, Delay2/1
  Out Frame Count/3(endOutFramem2) -> Delay4/1
  Dummy Frame Generator/5(headerEnd) -> dummyHeaderEnd/1
  Logical Operator8/1 -> nextFrameReady/1, Unit Delay Enabled Resettable Synchronous/2, Unit Delay Enabled Resettable Synchronous/1
  Logical Operator5/1 -> Logical Operator4/1
  Logical Operator9/1 -> Logical Operator8/2
  Logical Operator6/1 -> Logical Operator7/1
  Dummy Frame Generator/4(headerStart) -> dummyHeaderStart/1

== system Transmitter/PL Frame Gen/RAM FIFO/PL Header FIFO ==
  dataIn : Inport
  validIn : Inport  Port=2
  nextFrameReady : Inport  Port=3
  90x : MATLAB Function  TreatAsAtomicUnit=on
  Delay{1..3,9} (4 alike) : Delay  DelayLength=1
  HDL Counter2 : hdlsllib/Sources/HDL Counter  CountType=Count limited  CountInit=0  CountStep=1  CountMax=2^16 - 1  CountFromType=Initial value  CountFrom=0  CountResetPort=off  CountLoadPort=off  CountEnbPort=on  CountDirPort=off  CountHitOutputPort=off  CountDataType=Unsigned  CountWordLen=16  CountFracLen=0  CountSampTime=1
  HDL Counter3 : hdlsllib/Sources/HDL Counter  CountType=Count limited  CountInit=0  CountStep=1  CountMax=2^16 - 1  CountFromType=Initial value  CountFrom=0  CountResetPort=off  CountLoadPort=off  CountEnbPort=on  CountDirPort=off  CountHitOutputPort=off  CountDataType=Unsigned  CountWordLen=16  CountFracLen=0  CountSampTime=1
  Simple Dual Port RAM : hdlsllib/HDL RAMs/Simple Dual Port RAM  ram_size=16
  monostable 90x : Subsystem  Commented=on
  dataOut : Outport
  startOut : Outport  Port=2
  endOut : Outport  Port=3
  validOut : Outport  Port=4
  endOut1 : Outport  Port=5
  wires:
  dataIn/1 -> Simple Dual Port RAM/1
  validIn/1 -> Simple Dual Port RAM/3, HDL Counter2/1
  HDL Counter2/1 -> Simple Dual Port RAM/2
  nextFrameReady/1 -> 90x/1(trigger)
  90x/4(endOutm1) -> Delay3/1
  90x/1(validOut) -> HDL Counter3/1, Delay9/1
  90x/3(endOut) -> Delay2/1
  90x/2(startOut) -> Delay1/1
  Simple Dual Port RAM/1 -> dataOut/1
  HDL Counter3/1 -> Simple Dual Port RAM/4
  Delay9/1 -> validOut/1
  Delay1/1 -> startOut/1
  Delay2/1 -> endOut/1
  Delay3/1 -> endOut1/1

== system Transmitter/PL Frame Gen/RAM FIFO/Pilot Generator ==
  note: For debug purposes only
  trigger : Inport
  Multiply : Gain  Gain=2
  Pilot Block Length Valid Generator : Subsystem  Commented=on
  Pilot Block Length Valid Generator1 : MATLAB Function  TreatAsAtomicUnit=on
  Pilot or Unmodulated Carrier : Constant  Value=fi(exp(1i*pi/4),1,18,16)  SampleTime=1/Rsym
  dataOut : Outport
  endOut : Outport  Port=2
  validOut : Outport  Port=3
  endOut1 : Outport  Port=4
  wires:
  Multiply/1 -> dataOut/1
  Pilot or Unmodulated Carrier/1 -> Multiply/1
  trigger/1 -> Pilot Block Length Valid Generator1/1(trigger)
  Pilot Block Length Valid Generator1/1(endOut) -> endOut/1
  Pilot Block Length Valid Generator1/2(endOutm1) -> endOut1/1
  Pilot Block Length Valid Generator1/3(validOut) -> validOut/1

== system Transmitter/PL Frame Gen/DataStreamEnabler/monostable 8x/monostable ==
  In1 : Inport
  Compare To Constant : simulink/Logic and Bit Operations/Compare To Constant  relop===  const=8  OutDataTypeStr=boolean
  Compare To Constant1 : simulink/Logic and Bit Operations/Compare To Constant  relop=~=  const=0  OutDataTypeStr=boolean
  HDL Counter : hdlsllib/Sources/HDL Counter  CountType=Count limited  CountInit=0  CountStep=1  CountMax=8  CountFromType=Initial value  CountFrom=0  CountResetPort=on  CountLoadPort=off  CountEnbPort=on  CountDirPort=off  CountHitOutputPort=off  CountDataType=Unsigned  CountWordLen=8  CountFracLen=0  CountSampTime=1
  Logical Operator : Logic  Operator=OR  AllPortsSameDT=off  OutDataTypeStr=boolean
  Out1 : Outport
  wires:
  Compare To Constant1/1 -> Out1/1, Logical Operator/2
  HDL Counter/1 -> Compare To Constant1/1, Compare To Constant/1
  In1/1 -> Logical Operator/1
  Logical Operator/1 -> HDL Counter/2
  Compare To Constant/1 -> HDL Counter/1

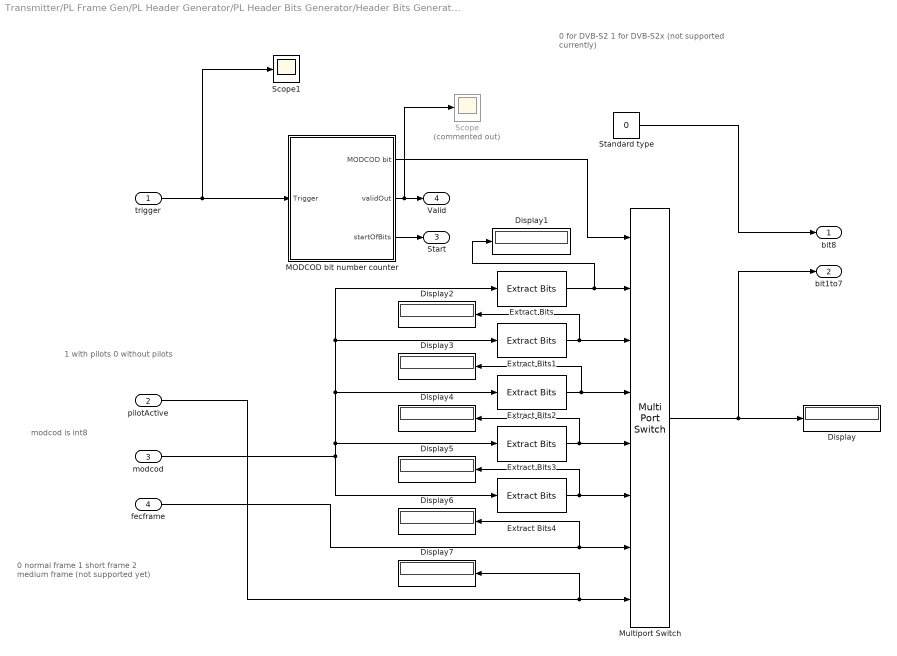
== system Transmitter/PL Frame Gen/PL Header Generator/PL Header Bits Generator/Header Bits Generator ==
  note: modcod is int8
  note: 0 for DVB-S2
      | 1 for DVB-S2x (not supported currently)
  note: 1 with pilots
      | 0 without pilots
  note: 0 normal frame
      | 1 short frame
      | 2 medium frame (not supported yet)
  trigger : Inport
  pilotActive : Inport  Port=2
  modcod : Inport  Port=3
  fecframe : Inport  Port=4
  Display{,1..7} (8 alike) : Display
  Extract Bits : simulink/Logic and Bit Operations/Extract Bits  bitsToExtract=Range of bits  numBits=8  bitIdxRange=0  outScalingMode=Treat bit field as an integer
  Extract Bits1 : simulink/Logic and Bit Operations/Extract Bits  bitsToExtract=Range of bits  numBits=8  bitIdxRange=1  outScalingMode=Treat bit field as an integer
  Extract Bits2 : simulink/Logic and Bit Operations/Extract Bits  bitsToExtract=Range of bits  numBits=8  bitIdxRange=2  outScalingMode=Treat bit field as an integer
  Extract Bits3 : simulink/Logic and Bit Operations/Extract Bits  bitsToExtract=Range of bits  numBits=8  bitIdxRange=3  outScalingMode=Treat bit field as an integer
  Extract Bits4 : simulink/Logic and Bit Operations/Extract Bits  bitsToExtract=Range of bits  numBits=8  bitIdxRange=4  outScalingMode=Treat bit field as an integer
  MODCOD bit number counter : Subsystem
  Multiport Switch : MultiPortSwitch  DataPortOrder=Zero-based contiguous  Inputs=7  zeroidx=on  SaturateOnIntegerOverflow=off  InputSameDT=off
  Scope : Scope  Commented=on
  Scope1 : Scope
  Standard type : Constant  Value=0  OutDataTypeStr=boolean  SampleTime=2/Rsym
  bit8 : Outport
  bit1to7 : Outport  Port=2
  Start : Outport  Port=3
  Valid : Outport  Port=4
  wires:
  trigger/1 -> Scope1/1, MODCOD bit number counter/1(Trigger)
  modcod/1 -> Extract Bits4/1, Extract Bits2/1, Extract Bits/1, Extract Bits1/1, Extract Bits3/1
  Extract Bits4/1 -> Display5/1, Multiport Switch/6
  Extract Bits3/1 -> Display4/1, Multiport Switch/5
  Extract Bits2/1 -> Display3/1, Multiport Switch/4
  Extract Bits1/1 -> Multiport Switch/3, Display2/1
  Extract Bits/1 -> Display1/1, Multiport Switch/2
  Multiport Switch/1 -> Display/1, bit1to7/1
  Standard type/1 -> bit8/1
  MODCOD bit number counter/3(startOfBits) -> Start/1
  MODCOD bit number counter/2(validOut) -> Scope/1, Valid/1
  fecframe/1 -> Display6/1, Multiport Switch/7
  MODCOD bit number counter/1(MODCOD bit) -> Multiport Switch/1
  pilotActive/1 -> Display7/1, Multiport Switch/8

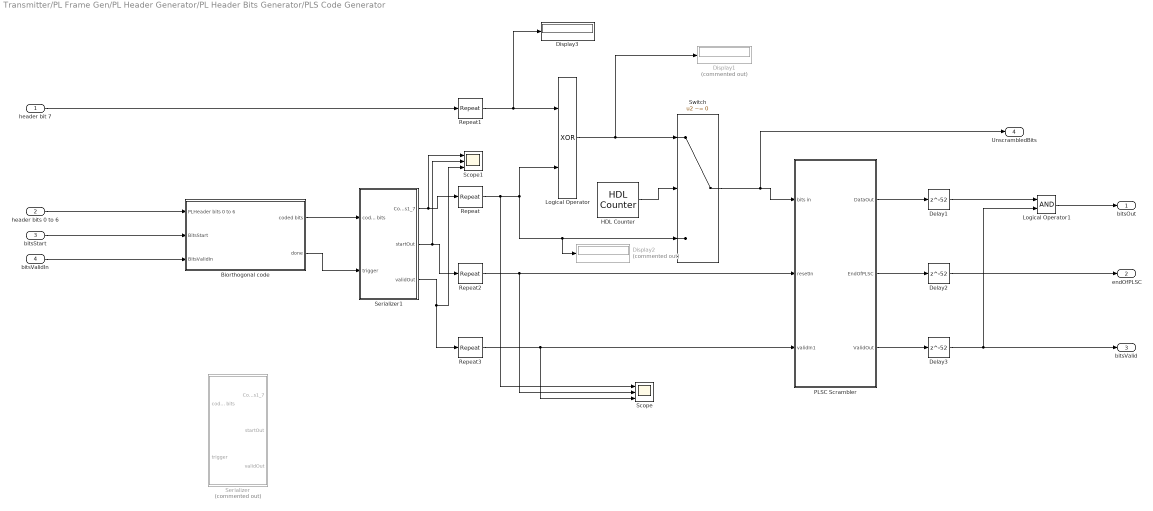
== system Transmitter/PL Frame Gen/PL Header Generator/PL Header Bits Generator/PLS Code Generator ==
  header bit 7 : Inport
  header bits 0 to 6 : Inport  Port=2
  bitsStart : Inport  Port=3
  bitsValidIn : Inport  Port=4
  Biorthogonal code : Subsystem
  Delay1 : Delay  DelayLength=52
  Delay2 : Delay  DelayLength=52
  Delay3 : Delay  DelayLength=52
  Display1 : Display  Commented=on
  Display2 : Display  Commented=on
  Display3 : Display
  HDL Counter : hdlsllib/Sources/HDL Counter  CountType=Count limited  CountInit=0  CountStep=1  CountMax=1  CountFromType=Initial value  CountFrom=0  CountResetPort=off  CountLoadPort=off  CountEnbPort=off  CountDirPort=off  CountHitOutputPort=off  CountDataType=Unsigned  CountWordLen=1  CountFracLen=0  CountSampTime=1/Rsym
  Logical Operator : Logic  Operator=XOR  AllPortsSameDT=off  OutDataTypeStr=boolean
  Logical Operator1 : Logic  AllPortsSameDT=off  OutDataTypeStr=boolean
  PLSC Scrambler : Subsystem
  Repeat{,1..3} (4 alike) : dspsigops/Repeat  N=2  RateOptions=Allow multirate processing  ic=0  mode=Unused parameter value
  Scope : Scope  NumInputPorts=3
  Scope1 : Scope  NumInputPorts=3
  Serializer : Subsystem  Commented=on
  Serializer1 : Subsystem
  Switch : Switch  Criteria=u2 ~= 0  SaturateOnIntegerOverflow=off  InputSameDT=off
  bitsOut : Outport
  endOfPLSC : Outport  Port=2
  bitsValid : Outport  Port=3
  UnscrambledBits : Outport  Port=4
  wires:
  header bits 0 to 6/1 -> Biorthogonal code/1(PLHeader bits 0 to 6)
  Serializer1/1(CodedBits1_7) -> Scope1/1, Repeat/1
  header bit 7/1 -> Repeat1/1
  Repeat/1 -> Scope/1, Switch/3, Display2/1, Logical Operator/2
  Repeat1/1 -> Display3/1, Logical Operator/1
  Logical Operator/1 -> Display1/1, Switch/1
  HDL Counter/1 -> Switch/2
  Switch/1 -> UnscrambledBits/1, PLSC Scrambler/1(bits in)
  PLSC Scrambler/1(DataOut) -> Delay1/1
  PLSC Scrambler/2(EndOfPLSC) -> Delay2/1
  PLSC Scrambler/3(ValidOut) -> Delay3/1
  bitsStart/1 -> Biorthogonal code/2(BitsStart)
  bitsValidIn/1 -> Biorthogonal code/3(BitsValidIn)
  Repeat2/1 -> Scope/2, PLSC Scrambler/2(resetIn)
  Serializer1/2(startOut) -> Scope1/2, Repeat2/1
  Serializer1/3(validOut) -> Scope1/3, Repeat3/1
  Repeat3/1 -> Scope/3, PLSC Scrambler/3(validIn1)
  Delay3/1 -> Logical Operator1/2, bitsValid/1
  Biorthogonal code/1(coded bits) -> Serializer1/1(coded bits)
  Biorthogonal code/2(done) -> Serializer1/2(trigger)
  Logical Operator1/1 -> bitsOut/1
  Delay2/1 -> endOfPLSC/1
  Delay1/1 -> Logical Operator1/1

== system Transmitter/PL Frame Gen/PL Header Generator/PL Header Bits Generator/SOF Generator ==
  note: Compensating for the delay in PLSCODE generator
  note: 1 for the duration of SOF (25 samples)
  note: Outputs one when the first bit of SOF sequence is passed
  note: valid flag
      | 1 if output of subsystem is valid
      | 0 if invalid
  note: The SOF sequence bits
  note: Trigger that enables the SOF Generator
  note: Actual SOF values
  note: Counter limited to 25 (SOF length)
  trigger : Inport
  Data Type Conversion : DataTypeConversion  OutDataTypeStr=boolean  SaturateOnIntegerOverflow=off  RndMeth=Floor
  Delay : Delay  DelayLength=42
  Delay1 : Delay  DelayLength=42
  Delay2 : Delay  DelayLength=42
  SOF Length Counter : Subsystem
  SOF Sequence : Lookup_n-D  NumberOfTableDimensions=1  BreakpointsSpecification=Even spacing  BreakpointsForDimension1=[-5:5]  BreakpointsForDimension1FirstPoint=0  Table=[0 1 1 0 0 0 1 1 0 1 0 0 1 0 1 1 1 0 1 0 0 0 0 0 1 0]  TableDataTypeStr=Inherit: Inherit from 'Table data'  InterpMethod=Flat  DiagnosticForOutOfRangeInput=Warning  InternalRulePriority=Speed  OutDataTypeStr=fixdt(0, 1, 0)  RndMeth=Simplest
  Upsample : dspsigops/Upsample  N=2  phase=0  RateOptions=Allow multirate processing  ic=0  mode=Unused parameter value
  dataOut : Outport
  validOut : Outport  Port=2
  startOfSOF : Outport  Port=3
  wires:
  SOF Sequence/1 -> Data Type Conversion/1
  SOF Length Counter/1(LUT address) -> SOF Sequence/1
  Data Type Conversion/1 -> Delay/1
  SOF Length Counter/2(validOut) -> Delay1/1
  SOF Length Counter/3(StartOfOSOF) -> Delay2/1
  trigger/1 -> Upsample/1
  Upsample/1 -> SOF Length Counter/1(Trigger)
  Delay/1 -> dataOut/1
  Delay1/1 -> validOut/1
  Delay2/1 -> startOfSOF/1
